simulink model "DCMG_3unit_multi_unit"  (R2018a)
settings: Solver=VariableStepAuto  StartTime=0.0  StopTime=4.2  FixedStep=0.1e-3  RelTol=1e-3
undefined symbols (not defined in the file): ALPHA, CAP, IND, k_ii_1, k_ii_2, k_ii_3, k_iv_1, k_iv_2, k_iv_3, k_pi_1, k_pi_2, k_pi_3, k_pv_1, k_pv_2, k_pv_3, n, P_load_inf, P_load_sup, r_jk, R_SK, rd1, rd2, rd3, tau, time1, time2, time3, V_ref, Zout_den_source, Zout_num_source
libraries: fl_lib x30, nesl_utility x22, elec_lib x6
settings Model: Creator=Marco  LastModifiedBy=carna
settings SolverCC: ZeroCrossAlgorithm=Adaptive
settings CodeAppCC: StateflowObjectComments=on
settings SimscapeCC: SimscapeNormalizeSystem=off

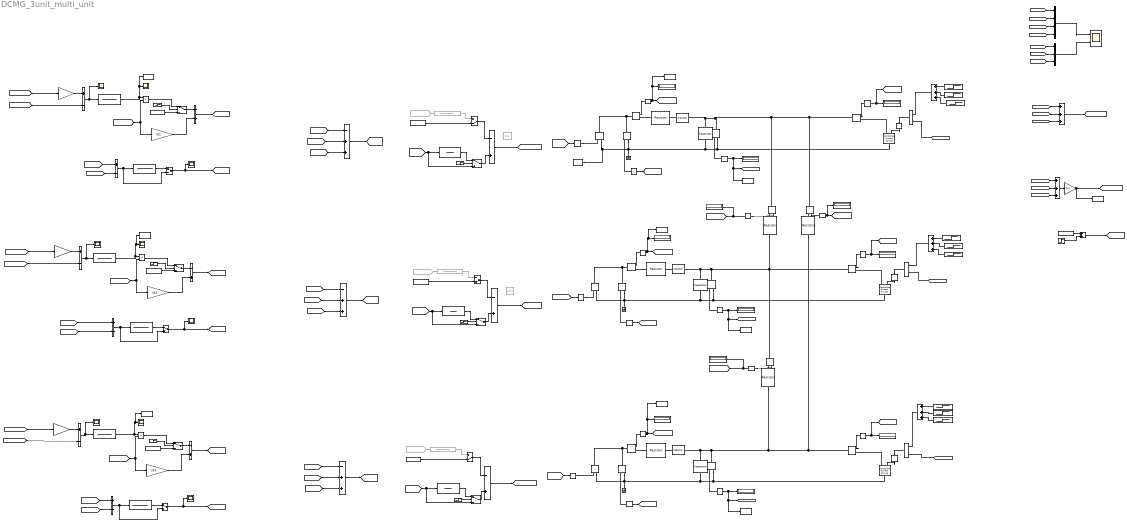
== system DCMG_3unit_multi_unit ==
  note: V MG
  note: I MG
  note: Delta v 1
  note: DELTA I
  note: Delta R droop
  note: Delta v 2
  note: DELTA I
  note: Delta R droop
  note: Delta v 3
  note: DELTA I
  note: Delta R droop
  Add{1..2,5,7,10,12} (6 alike) : Sum  Inputs=+-
  Add{4,6,9,11,13,17} (6 alike) : Sum  Inputs=-+
  Add14 : Sum  Inputs=-++
  Add{15..16,18..19,22} (5 alike) : Sum  Inputs=+++
  Add3 : Sum  Inputs=-++
  Add46 : Sum
  Add8 : Sum  Inputs=-++
  C bus 1 : elec_lib/Passive Devices/Capacitor  enable_table=0  c=CAP(1) F  Cvec=[1.0e-5, 1.0e-6] F  Vvec=[0.0, 10.0] V  CV_table_symmetry=1  C_tol=5  enable_C_tol=0  tol_distribution=1  nSigma=4  r=1e-6 Ohm  g=0 1/Ohm  enable_operating_limits=0  operating_limit_action=2  max_working_voltage_range=[-25.0, 25.0] V  power_rating=1 W  enable_faults=0  fault_action=1  Cscale_faulted=100  R_faulted=1e-3 Ohm  G_faulted=0 1/Ohm  tau_fault=1e-3 s  enable_temporal_fault=0  t_fault=1 s  enable_behavioral_fault=0  max_permissible_voltage_range=[-100.0, 100.0] V  t_fail_on_voltage=1 s  i_specify=off  i_priority=None  i=0 A  i_nominal_specify=off  i_nominal_unit=A  i_nominal_value=1  v_specify=off  v_priority=None  v=0 V  v_nominal_specify=off  v_nominal_unit=V  v_nominal_value=1  vc_specify=off  vc_priority=High  vc=0 V  vc_nominal_specify=off  vc_nominal_unit=V  vc_nominal_value=1
  C bus 2 : elec_lib/Passive Devices/Capacitor  enable_table=0  c=CAP(2) F  Cvec=[1.0e-5, 1.0e-6] F  Vvec=[0.0, 10.0] V  CV_table_symmetry=1  C_tol=5  enable_C_tol=0  tol_distribution=1  nSigma=4  r=1e-6 Ohm  g=0 1/Ohm  enable_operating_limits=0  operating_limit_action=2  max_working_voltage_range=[-25.0, 25.0] V  power_rating=1 W  enable_faults=0  fault_action=1  Cscale_faulted=100  R_faulted=1e-3 Ohm  G_faulted=0 1/Ohm  tau_fault=1e-3 s  enable_temporal_fault=0  t_fault=1 s  enable_behavioral_fault=0  max_permissible_voltage_range=[-100.0, 100.0] V  t_fail_on_voltage=1 s  i_specify=off  i_priority=None  i=0 A  i_nominal_specify=off  i_nominal_unit=A  i_nominal_value=1  v_specify=off  v_priority=None  v=0 V  v_nominal_specify=off  v_nominal_unit=V  v_nominal_value=1  vc_specify=off  vc_priority=High  vc=0 V  vc_nominal_specify=off  vc_nominal_unit=V  vc_nominal_value=1
  C bus 3 : elec_lib/Passive Devices/Capacitor  enable_table=0  c=CAP(3) F  Cvec=[1.0e-5, 1.0e-6] F  Vvec=[0.0, 10.0] V  CV_table_symmetry=1  C_tol=5  enable_C_tol=0  tol_distribution=1  nSigma=4  r=1e-6 Ohm  g=0 1/Ohm  enable_operating_limits=0  operating_limit_action=2  max_working_voltage_range=[-25.0, 25.0] V  power_rating=1 W  enable_faults=0  fault_action=1  Cscale_faulted=100  R_faulted=1e-3 Ohm  G_faulted=0 1/Ohm  tau_fault=1e-3 s  enable_temporal_fault=0  t_fault=1 s  enable_behavioral_fault=0  max_permissible_voltage_range=[-100.0, 100.0] V  t_fail_on_voltage=1 s  i_specify=off  i_priority=None  i=0 A  i_nominal_specify=off  i_nominal_unit=A  i_nominal_value=1  v_specify=off  v_priority=None  v=0 V  v_nominal_specify=off  v_nominal_unit=V  v_nominal_value=1  vc_specify=off  vc_priority=High  vc=0 V  vc_nominal_specify=off  vc_nominal_unit=V  vc_nominal_value=1
  Close loop equivalent1 : TransferFcn  Numerator=[k_pv_1 k_iv_1 ]  Denominator=[1 0]
  Close loop equivalent10 : TransferFcn  Numerator=[1 ]  Denominator=[tau 1]
  Close loop equivalent2 : TransferFcn  Numerator=[1 ]  Denominator=[tau 1]
  Close loop equivalent3 : TransferFcn  Numerator=[k_pv_2 k_iv_2 ]  Denominator=[1 0]
  Close loop equivalent4 : TransferFcn  Commented=on  Numerator=Zout_num_source  Denominator=Zout_den_source
  Close loop equivalent6 : TransferFcn  Commented=on  Numerator=Zout_num_source  Denominator=Zout_den_source
  Close loop equivalent7 : TransferFcn  Numerator=[k_pv_3 k_iv_3 ]  Denominator=[1 0]
  Close loop equivalent8 : TransferFcn  Commented=on  Numerator=Zout_num_source  Denominator=Zout_den_source
  Close loop equivalent9 : TransferFcn  Numerator=[1 ]  Denominator=[tau 1]
  Constant{3,8,10,15..16,18} (6 alike) : Constant  Value=0
  Constant4 : Constant  Value=V_ref
  Controlled Current Source5 : fl_lib/Electrical/Electrical Sources/Controlled Current Source
  Controlled Current Source6 : fl_lib/Electrical/Electrical Sources/Controlled Current Source
  Controlled Current Source7 : fl_lib/Electrical/Electrical Sources/Controlled Current Source
  Controlled Voltage Source : fl_lib/Electrical/Electrical Sources/Controlled Voltage Source
  Controlled Voltage Source1 : fl_lib/Electrical/Electrical Sources/Controlled Voltage Source
  Controlled Voltage Source3 : fl_lib/Electrical/Electrical Sources/Controlled Voltage Source
  Current cloop transfer- Transport Delay2 : TransportDelay  Commented=on  DelayTime=0.1e-3
  Current cloop transfer- Transport Delay3 : TransportDelay  Commented=on  DelayTime=0.1e-3
  Current load 1 : fl_lib/Electrical/Electrical Sensors/Current Sensor
  Current load 2 : fl_lib/Electrical/Electrical Sensors/Current Sensor
  Current load 3 : fl_lib/Electrical/Electrical Sensors/Current Sensor
  Current output {1..6} (6 alike) : fl_lib/Electrical/Electrical Sensors/Current Sensor
  Display{,1..11} (12 alike) : Display
  Divide3 : Product  Inputs=*/
  Divide4 : Product  Inputs=*/
  Divide5 : Product  Inputs=*/
  Electrical Reference : fl_lib/Electrical/Electrical Elements/Electrical Reference
  Electrical Reference1 : fl_lib/Electrical/Electrical Elements/Electrical Reference
  Electrical Reference2 : fl_lib/Electrical/Electrical Elements/Electrical Reference
  From17 : From  Commented=on  GotoTag=io_source_2
  From26 : From  Commented=on  GotoTag=io_source_1
  From29 : From  Commented=on  GotoTag=io_source_3
  Gain1 : Gain  Gain=ALPHA(1,1)
  Gain2 : Gain  Gain=rd1
  Gain3 : Gain  Gain=ALPHA(2,2)
  Gain4 : Gain  Gain=rd2
  Gain5 : Gain  Gain=1/n
  Gain6 : Gain  Gain=ALPHA(3,3)
  Gain7 : Gain  Gain=rd3
  L serie 1 : elec_lib/Passive Devices/Inductor  l=IND(1) H  L_tol=20  enable_L_tol=0  tol_distribution=1  nSigma=4  r=0 Ohm  g=1e-9 1/Ohm  enable_operating_limits=0  operating_limit_action=2  max_working_current=1 A  power_rating=1 W  enable_faults=0  fault_action=1  lambdaPercent=50  k_faulted=0.9999  turnsShort=0  openCct=0  groundShort=0  groundShortG=0 1/Ohm  tau_fault=1e-3 s  enable_temporal_fault=0  t_fault=1 s  enable_behavioral_fault=0  max_permissible_voltage=100 V  n_fail_on_voltage=1  max_permissible_current=1 A  t_fail_on_current=1 s  i_L_specify=off  i_L_priority=High  i_L=0 A  i_L_nominal_specify=off  i_L_nominal_unit=A  i_L_nominal_value=1
      settings: SourceProductName=Simscape Electronics  SourceProductBaseCode=SN
  L serie 2 : elec_lib/Passive Devices/Inductor  l=IND(2) H  L_tol=20  enable_L_tol=0  tol_distribution=1  nSigma=4  r=0 Ohm  g=1e-9 1/Ohm  enable_operating_limits=0  operating_limit_action=2  max_working_current=1 A  power_rating=1 W  enable_faults=0  fault_action=1  lambdaPercent=50  k_faulted=0.9999  turnsShort=0  openCct=0  groundShort=0  groundShortG=0 1/Ohm  tau_fault=1e-3 s  enable_temporal_fault=0  t_fault=1 s  enable_behavioral_fault=0  max_permissible_voltage=100 V  n_fail_on_voltage=1  max_permissible_current=1 A  t_fail_on_current=1 s  i_L_specify=off  i_L_priority=High  i_L=0 A  i_L_nominal_specify=off  i_L_nominal_unit=A  i_L_nominal_value=1
      settings: SourceProductName=Simscape Electronics  SourceProductBaseCode=SN
  L serie 3 : elec_lib/Passive Devices/Inductor  l=IND(3) H  L_tol=20  enable_L_tol=0  tol_distribution=1  nSigma=4  r=0 Ohm  g=1e-9 1/Ohm  enable_operating_limits=0  operating_limit_action=2  max_working_current=1 A  power_rating=1 W  enable_faults=0  fault_action=1  lambdaPercent=50  k_faulted=0.9999  turnsShort=0  openCct=0  groundShort=0  groundShortG=0 1/Ohm  tau_fault=1e-3 s  enable_temporal_fault=0  t_fault=1 s  enable_behavioral_fault=0  max_permissible_voltage=100 V  n_fail_on_voltage=1  max_permissible_current=1 A  t_fail_on_current=1 s  i_L_specify=off  i_L_priority=High  i_L=0 A  i_L_nominal_specify=off  i_L_nominal_unit=A  i_L_nominal_value=1
      settings: SourceProductName=Simscape Electronics  SourceProductBaseCode=SN
  Manual Switch1 : ManualSwitch
  Manual Switch10 : ManualSwitch  CurrentSetting=0
  Manual Switch2 : ManualSwitch  CurrentSetting=0
  Manual Switch5 : ManualSwitch
  Manual Switch6 : ManualSwitch  CurrentSetting=0
  Manual Switch7 : ManualSwitch
  Mux : Mux  Inputs=3
  Mux1 : Mux
  PI i : TransferFcn  Numerator=[k_pi_1 k_ii_1 ]  Denominator=[1 0]
  PI i 2 : TransferFcn  Numerator=[k_pi_2 k_ii_2 ]  Denominator=[1 0]
  PI i2 : TransferFcn  Numerator=[k_pi_3 k_ii_3 ]  Denominator=[1 0]
  PS-Simulink Converter{,1..8,11..16} (15 alike) : nesl_utility/PS-Simulink Converter  PhysicalDomain=network_engine_domain  SubClassName=ps_output  LeftPortType=input  RightPortType=output  PseudoPeriodic=off  Frequencies=[]  Unit=1  AffineConversion=off
  Product : Product
  Product1 : Product
  Product7 : Product
  R serie 1 : fl_lib/Electrical/Electrical Elements/Resistor  R=R_SK(1,1) Ohm  i_specify=off  i_priority=None  i=0 A  i_nominal_specify=off  i_nominal_unit=A  i_nominal_value=1  v_specify=off  v_priority=None  v=0 V  v_nominal_specify=off  v_nominal_unit=V  v_nominal_value=1
  R serie 12 : fl_lib/Electrical/Electrical Elements/Resistor  R=r_jk Ohm  i_specify=off  i_priority=None  i=0 A  i_nominal_specify=off  i_nominal_unit=A  i_nominal_value=1  v_specify=off  v_priority=None  v=0 V  v_nominal_specify=off  v_nominal_unit=V  v_nominal_value=1
  R serie 13 : fl_lib/Electrical/Electrical Elements/Resistor  R=r_jk Ohm  i_specify=off  i_priority=None  i=0 A  i_nominal_specify=off  i_nominal_unit=A  i_nominal_value=1  v_specify=off  v_priority=None  v=0 V  v_nominal_specify=off  v_nominal_unit=V  v_nominal_value=1
  R serie 2 : fl_lib/Electrical/Electrical Elements/Resistor  R=R_SK(2,2) Ohm  i_specify=off  i_priority=None  i=0 A  i_nominal_specify=off  i_nominal_unit=A  i_nominal_value=1  v_specify=off  v_priority=None  v=0 V  v_nominal_specify=off  v_nominal_unit=V  v_nominal_value=1
  R serie 23 : fl_lib/Electrical/Electrical Elements/Resistor  R=r_jk Ohm  i_specify=off  i_priority=None  i=0 A  i_nominal_specify=off  i_nominal_unit=A  i_nominal_value=1  v_specify=off  v_priority=None  v=0 V  v_nominal_specify=off  v_nominal_unit=V  v_nominal_value=1
  R serie 3 : fl_lib/Electrical/Electrical Elements/Resistor  R=R_SK(3,3) Ohm  i_specify=off  i_priority=None  i=0 A  i_nominal_specify=off  i_nominal_unit=A  i_nominal_value=1  v_specify=off  v_priority=None  v=0 V  v_nominal_specify=off  v_nominal_unit=V  v_nominal_value=1
  Scope : Scope  NumInputPorts=2
  Scope{1..9} (9 alike) : Scope
  Simulink-PS Converter{,1,8..11} (6 alike) : nesl_utility/Simulink-PS Converter  PhysicalDomain=network_engine_domain  SubClassName=ps_input  LeftPortType=input  RightPortType=output  PseudoPeriodic=off  Frequencies=[]  NoiseDistribution=none  NoiseParameters=[]  Unit=1  AffineConversion=off  FilteringAndDerivatives=provide  SimscapeFilterOrder=1  InputFilterTimeConstant=0.001  UdotUserProvided=0
  Solver Configuration : nesl_utility/Solver Configuration  PhysicalDomain=network_engine_domain  SubClassName=solver  LeftPortType=input  RightPortType=generic  Tones=[]  Harmonics=[]  SimulateNoise=off  Profile=off  UseLocalSampling=off  EnableSwitchedLinearOptims=on  FrequencyDomain=off  UseCCode=off  RelTol=0.001  AbsTol=1e-06  MinStep=1e-09  ToWorkspace=off  RevertToSquareIcSolve=off  NumHomotopyIterations=100  PhasorMode=off  PhasorModeNumHarmonics=1  DoDC=off  ResidualTolerance=1e-09  UseLocalSolver=off  LocalSolverChoice=NE_BACKWARD_EULER_ADVANCER  LocalSolverSampleTime=0.001  DoFixedCost=off  MaxNonlinIter=3  MaxModeIter=2  LinearAlgebra=Sparse  EquationFormulation=NE_TIME_EF  DelaysMemoryBudget=1024  AutomaticFiltering=on  FilteringTimeConstant=0.001
  Step1 : Step  Time=0  SampleTime=0
  Step12 : Step  Time=0.5  SampleTime=0
  Step13 : Step  Time=time3  After=-0.1*P_load_inf(3)  SampleTime=0
  Step14 : Step  Time=0  SampleTime=0
  Step15 : Step  Time=time1  After=P_load_inf(1)  SampleTime=0
  Step17 : Step  Time=time2  After=-100  SampleTime=0
  Step2 : Step  Time=0  SampleTime=0
  Step3 : Step  Time=time2  After=P_load_sup(1)-P_load_inf(1)  SampleTime=0
  Step31 : Step  Time=time2  After=P_load_sup(3)-P_load_inf(3)  SampleTime=0
  Step32 : Step  Time=time3  After=-0.1*P_load_inf(1)  SampleTime=0
  Step37 : Step  Time=time1  After=P_load_inf(2)  SampleTime=0
  Step38 : Step  Time=time3  After=-0.1*P_load_inf(2)  SampleTime=0
  Step39 : Step  Time=time2  After=P_load_sup(2)-P_load_inf(2)  SampleTime=0
  Step4 : Step  Time=0.5  SampleTime=0
  Step6 : Step  Time=0.5  SampleTime=0
  Step8 : Step  Time=time1  After=P_load_inf(3)  SampleTime=0
  Switch : Switch  Criteria=u2 > Threshold  Threshold=0.5
  Switch1 : Switch  Criteria=u2 > Threshold
  Switch2 : Switch  Criteria=u2 > Threshold
  Switch3 : Switch  Criteria=u2 > Threshold
  Switch4 : Switch  Criteria=u2 > Threshold  Threshold=0.5
  Switch5 : Switch  Criteria=u2 > Threshold  Threshold=0.5
  To Workspace : ToWorkspace  VariableName=i_1_sa  SaveFormat=Timeseries  SampleTime=-1
  To Workspace1 : ToWorkspace  VariableName=i_2_sa  SaveFormat=Timeseries  SampleTime=-1
  To Workspace2 : ToWorkspace  VariableName=i_3_sa  SaveFormat=Timeseries  SampleTime=-1
  To Workspace3 : ToWorkspace  VariableName=v_b1_sa  SaveFormat=Timeseries  SampleTime=-1
  To Workspace4 : ToWorkspace  VariableName=v_b2_sa  SaveFormat=Timeseries  SampleTime=-1
  To Workspace5 : ToWorkspace  VariableName=v_b3_sa  SaveFormat=Timeseries  SampleTime=-1
  To Workspace6 : ToWorkspace  VariableName=deltaR1_sa  SaveFormat=Timeseries  SampleTime=-1
  To Workspace7 : ToWorkspace  VariableName=deltaR2_sa  SaveFormat=Timeseries  SampleTime=-1
  To Workspace8 : ToWorkspace  VariableName=deltaR3_sa  SaveFormat=Timeseries  SampleTime=-1
  To Workspace9 : ToWorkspace  VariableName=V_MG_sa  SaveFormat=Timeseries  SampleTime=-1
  Voltage bus 1 : fl_lib/Electrical/Electrical Sensors/Voltage Sensor
  Voltage bus 2 : fl_lib/Electrical/Electrical Sensors/Voltage Sensor
  Voltage bus 3 : fl_lib/Electrical/Electrical Sensors/Voltage Sensor
  Voltage output 1 : fl_lib/Electrical/Electrical Sensors/Voltage Sensor
  Voltage output 2 : fl_lib/Electrical/Electrical Sensors/Voltage Sensor
  Voltage output 3 : fl_lib/Electrical/Electrical Sensors/Voltage Sensor
  wires:
  PS-Simulink Converter/1 -> To Workspace/1, Display2/1, [io_source_1]
  PS-Simulink Converter5/1 -> [i_cpl_1], Display/1
  PS-Simulink Converter4/1 -> To Workspace3/1, [v_bus_1], Display1/1
  Mux1/1 -> Scope/1
  [V_out2] -> Mux1/2
  [V_out1] -> Mux1/1
  [io_source_1] -> Mux/1
  [io_source_2] -> Mux/2
  Mux/1 -> Scope/2
  PS-Simulink Converter1/1 -> [V_out1]
  [V_out_source_1] -> Simulink-PS Converter/1
  Add13/1 -> [V_out_source_1]
  Add3/1 -> [V_ref_tot_1]
  [V_REF_c] -> Add3/2
  [V_REF_c] -> Add1/1
  [io_source_1] -> Add2/2
  Gain1/1 -> Add2/1
  Add2/1 -> Scope1/1, PI i/1
  PI i/1 -> To Workspace6/1, Scope2/1, Product/1
  [io_source_1] -> Gain2/1, Product/2
  [delta_I_1] -> Add3/1
  [delta_V_1] -> Add3/3
  Constant8/1 -> Switch1/3
  Switch1/1 -> Add4/1
  Product/1 -> Switch1/1
  Gain2/1 -> Add4/2
  Manual Switch5/1 -> Scope5/1, [delta_V_1]
  Close loop equivalent1/1 -> Manual Switch5/1
  Add1/1 -> Close loop equivalent1/1, Manual Switch5/2
  Step2/1 -> Switch1/2
  [V_MG] -> Add1/2
  [i_MG] -> Gain1/1
  From26/1 -> Close loop equivalent6/1
  Manual Switch6/1 -> Add13/1
  Close loop equivalent6/1 -> Manual Switch6/1
  Constant15/1 -> Manual Switch6/2
  Divide3/1 -> Simulink-PS Converter8/1
  Divide4/1 -> Simulink-PS Converter10/1
  [V_out_source_2] -> Simulink-PS Converter9/1
  PS-Simulink Converter12/1 -> [V_out2]
  PS-Simulink Converter14/1 -> Display7/1, [i_cpl_2]
  PS-Simulink Converter11/1 -> [io_source_2], To Workspace1/1, Display9/1
  PS-Simulink Converter2/1 -> To Workspace2/1, Display11/1, [io_source_3]
  PS-Simulink Converter16/1 -> [i_cpl_3], Display3/1
  PS-Simulink Converter15/1 -> To Workspace5/1, [v_bus_3], Display10/1
  PS-Simulink Converter3/1 -> [V_out3]
  [V_out_source_3] -> Simulink-PS Converter11/1
  Divide5/1 -> Simulink-PS Converter1/1
  Add4/1 -> [delta_I_1]
  Add9/1 -> [delta_I_2]
  [V_ref_tot_2] -> Switch/3, Close loop equivalent2/1
  Switch/1 -> Add6/2
  Constant3/1 -> Manual Switch2/2
  Close loop equivalent4/1 -> Manual Switch2/1
  Manual Switch2/1 -> Add6/1
  From17/1 -> Close loop equivalent4/1
  [i_MG] -> Gain3/1
  [V_MG] -> Add5/2
  Step1/1 -> Switch2/2
  Add5/1 -> Manual Switch1/2, Close loop equivalent3/1
  Close loop equivalent3/1 -> Manual Switch1/1
  Manual Switch1/1 -> Scope6/1, [delta_V_2]
  Gain4/1 -> Add9/2
  Product1/1 -> Switch2/1
  Switch2/1 -> Add9/1
  Constant10/1 -> Switch2/3
  [delta_V_2] -> Add8/3
  [delta_I_2] -> Add8/1
  [io_source_2] -> Product1/2, Gain4/1
  PI i 2/1 -> Product1/1, To Workspace7/1, Scope4/1
  Add7/1 -> Scope3/1, PI i 2/1
  Gain3/1 -> Add7/1
  [io_source_2] -> Add7/2
  [V_REF_c] -> Add5/1
  [V_REF_c] -> Add8/2
  Add8/1 -> [V_ref_tot_2]
  Add6/1 -> [V_out_source_2]
  Add14/1 -> [V_ref_tot_3]
  [V_REF_c] -> Add14/2
  [V_REF_c] -> Add10/1
  [io_source_3] -> Add12/2
  Gain6/1 -> Add12/1
  Add12/1 -> Scope7/1, PI i2/1
  PI i2/1 -> To Workspace8/1, Scope9/1, Product7/1
  [io_source_3] -> Gain7/1, Product7/2
  [delta_I_3] -> Add14/1
  [delta_V_3] -> Add14/3
  Constant16/1 -> Switch3/3
  Switch3/1 -> Add17/1
  Product7/1 -> Switch3/1
  Gain7/1 -> Add17/2
  Manual Switch7/1 -> Scope8/1, [delta_V_3]
  Close loop equivalent7/1 -> Manual Switch7/1
  Add10/1 -> Close loop equivalent7/1, Manual Switch7/2
  Step14/1 -> Switch3/2
  [V_MG] -> Add10/2
  [i_MG] -> Gain6/1
  From29/1 -> Close loop equivalent8/1
  Manual Switch10/1 -> Add11/1
  Close loop equivalent8/1 -> Manual Switch10/1
  Constant18/1 -> Manual Switch10/2
  Switch5/1 -> Add11/2
  Add17/1 -> [delta_I_3]
  [i_cpl_1] -> Add15/1
  [i_cpl_2] -> Add15/2
  [i_cpl_3] -> Add15/3
  [v_bus_1] -> Add16/1
  [v_bus_2] -> Add16/2
  [v_bus_3] -> Add16/3
  Add16/1 -> Gain5/1
  [io_source_3] -> Mux/3
  [V_MG] -> Mux1/4
  [V_out3] -> Mux1/3
  PS-Simulink Converter6/1 -> Display4/1, [i_bus_2_3]
  PS-Simulink Converter7/1 -> Display5/1, [i_bus_1_2]
  PS-Simulink Converter8/1 -> Display6/1, [i_bus_1_3]
  Add11/1 -> [V_out_source_3]
  PS-Simulink Converter13/1 -> Display8/1, To Workspace4/1, [v_bus_2]
  Add46/1 -> [V_REF_c]
  Constant4/1 -> Add46/1
  Step17/1 -> Add46/2
  [v_bus_3] -> Divide5/2
  [v_bus_2] -> Divide4/2
  [v_bus_1] -> Divide3/2
  Gain5/1 -> [V_MG], To Workspace9/1
  Add15/1 -> [i_MG]
  Step4/1 -> Switch/2
  Close loop equivalent2/1 -> Switch/1
  Step6/1 -> Switch4/2
  Close loop equivalent9/1 -> Switch4/1
  Switch4/1 -> Add13/2
  [V_ref_tot_1] -> Switch4/3, Close loop equivalent9/1
  Step12/1 -> Switch5/2
  Close loop equivalent10/1 -> Switch5/1
  [V_ref_tot_3] -> Switch5/3, Close loop equivalent10/1
  Add18/1 -> Divide4/1
  Step37/1 -> Add18/1
  Step39/1 -> Add18/2
  Step38/1 -> Add18/3
  Step32/1 -> Add22/3
  Step3/1 -> Add22/2
  Step15/1 -> Add22/1
  Add22/1 -> Divide3/1
  Step13/1 -> Add19/3
  Step31/1 -> Add19/2
  Step8/1 -> Add19/1
  Add19/1 -> Divide5/1
  connections:
  Controlled Voltage Source/LConn1 -- Current output 1/LConn1 -- Voltage output 1/LConn1
  Current load 1/RConn1 -- PS-Simulink Converter5/LConn1
  PS-Simulink Converter4/LConn1 -- Voltage bus 1/RConn1
  PS-Simulink Converter1/LConn1 -- Voltage output 1/RConn1
  Simulink-PS Converter/RConn1 -- Controlled Voltage Source/RConn1
  R serie 1/LConn1 -- Current output 1/RConn2
  PS-Simulink Converter/LConn1 -- Current output 1/RConn1
  Controlled Voltage Source/RConn2 -- Voltage bus 1/RConn2 -- Controlled Current Source5/LConn1 -- C bus 1/RConn1 -- Voltage output 1/RConn2 -- Electrical Reference/LConn1 -- Solver Configuration/RConn1
  L serie 1/LConn1 -- R serie 1/RConn1
  C bus 1/LConn1 -- Current output 6/LConn1 -- Current load 1/LConn1 -- Current output 4/LConn1 -- Voltage bus 1/LConn1 -- L serie 1/RConn1
  Controlled Current Source5/RConn2 -- Current load 1/RConn2
  Simulink-PS Converter8/RConn1 -- Controlled Current Source5/RConn1
  Controlled Voltage Source3/LConn1 -- Voltage output 2/LConn1 -- Current output 2/LConn1
  Voltage bus 2/RConn2 -- Controlled Current Source6/LConn1 -- C bus 2/RConn1 -- Controlled Voltage Source3/RConn2 -- Electrical Reference1/LConn1 -- Voltage output 2/RConn2
  Current load 2/LConn1 -- Current output 5/LConn1 -- R serie 12/RConn1 -- Voltage bus 2/LConn1 -- C bus 2/LConn1 -- L serie 2/RConn1
  Simulink-PS Converter10/RConn1 -- Controlled Current Source6/RConn1
  Controlled Current Source6/RConn2 -- Current load 2/RConn2
  L serie 2/LConn1 -- R serie 2/RConn1
  PS-Simulink Converter11/LConn1 -- Current output 2/RConn1
  R serie 2/LConn1 -- Current output 2/RConn2
  PS-Simulink Converter13/LConn1 -- Voltage bus 2/RConn1
  PS-Simulink Converter12/LConn1 -- Voltage output 2/RConn1
  Simulink-PS Converter9/RConn1 -- Controlled Voltage Source3/RConn1
  Current load 2/RConn1 -- PS-Simulink Converter14/LConn1
  Voltage output 3/LConn1 -- Controlled Voltage Source1/LConn1 -- Current output 3/LConn1
  Controlled Current Source7/LConn1 -- Voltage output 3/RConn2 -- Electrical Reference2/LConn1 -- Controlled Voltage Source1/RConn2 -- C bus 3/RConn1 -- Voltage bus 3/RConn2
  Voltage bus 3/LConn1 -- R serie 13/RConn1 -- Current load 3/LConn1 -- R serie 23/RConn1 -- L serie 3/RConn1 -- C bus 3/LConn1
  Current load 3/RConn1 -- PS-Simulink Converter16/LConn1
  PS-Simulink Converter3/LConn1 -- Voltage output 3/RConn1
  Simulink-PS Converter11/RConn1 -- Controlled Voltage Source1/RConn1
  PS-Simulink Converter15/LConn1 -- Voltage bus 3/RConn1
  R serie 3/LConn1 -- Current output 3/RConn2
  L serie 3/LConn1 -- R serie 3/RConn1
  Simulink-PS Converter1/RConn1 -- Controlled Current Source7/RConn1
  PS-Simulink Converter2/LConn1 -- Current output 3/RConn1
  Controlled Current Source7/RConn2 -- Current load 3/RConn2
  Current output 4/RConn2 -- R serie 12/LConn1
  Current output 5/RConn2 -- R serie 23/LConn1
  Current output 6/RConn2 -- R serie 13/LConn1
  PS-Simulink Converter6/LConn1 -- Current output 5/RConn1
  PS-Simulink Converter7/LConn1 -- Current output 4/RConn1
  Current output 6/RConn1 -- PS-Simulink Converter8/LConn1
